simulink model "test_equalizer"  (Simulink 7.4)
settings: Solver=ode45  StartTime=0  StopTime=100  RelTol=1e-3
libraries: xbsIndex_r4 x7, casper_library x2, xps_library x1, isi_correlator_lib x1
settings Model: Creator=wjm  LastModifiedBy=wjm
settings OptimizationCC: InitFltsAndDblsToZero=on

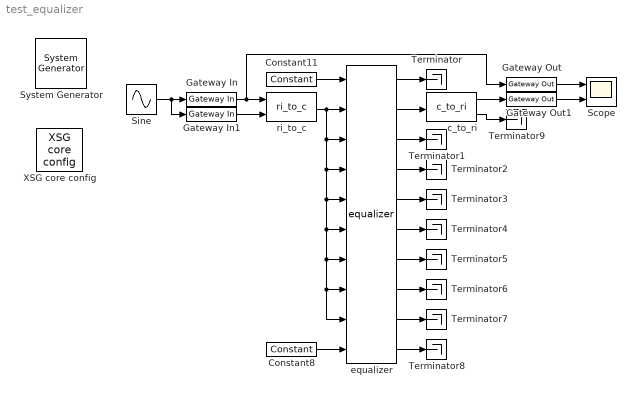
== system test_equalizer ==
  " System Generator" : xbsIndex_r4/ System Generator  Tag=genX  SystemSampleTime=-1  xilinxfamily=virtex5  part=xc5vsx95t  speed=-1  package=ff1136  synthesis_tool=XST  clock_wrapper=Clock Enables  directory=./isi_spectrometer/sysgen  testbench=off  simulink_period=1  sysclk_period=5  dcm_input_clock_period=100  incr_netlist=off  trim_vbits=Everywhere in SubSystem  dbl_ovrd=According to Block Masks  core_generation=According to Block Masks  run_coregen=off  deprecated_control=off  eval_field=0  block_type=sysgen
      settings: block_version=10.1.1
  Constant11 : xbsIndex_r4/Constant  arith_type=Boolean  const=0  n_bits=1  bin_pt=0  explicit_period=on  period=1  equ=P=C  opselect=C  inp2=PCIN>>17  opr=+  inp1=P  carry=CIN  dbl_ovrd=off  block_type=constant
      settings: block_version=10.1.1
  Constant8 : xbsIndex_r4/Constant  arith_type=Unsigned  const=1  n_bits=4  bin_pt=0  explicit_period=on  period=1  equ=P=C  opselect=C  inp2=PCIN>>17  opr=+  inp1=P  carry=CIN  dbl_ovrd=off  block_type=constant
      settings: block_version=10.1.1
  Gateway In : xbsIndex_r4/Gateway In  arith_type="Signed  (2's comp)"  n_bits=8  bin_pt=7  quantization="Round  (unbiased: +/- Inf)"  overflow=Wrap  period=1  dbl_ovrd=off  timing_constraint=None  locs_specified=off  LOCs={}  hdl_port=on  block_type=gatewayin
      settings: infoedit="Gateway in block.  Converts inputs of type Simulink integer, double and fixed point to  Xilinx fixed point type.<br><br>Hardware notes:  In hardware these blocks become top level input ports."  block_version=10.1.3
  Gateway In1 : xbsIndex_r4/Gateway In  arith_type="Signed  (2's comp)"  n_bits=8  bin_pt=7  quantization=Truncate  overflow=Wrap  period=1  dbl_ovrd=off  timing_constraint=None  locs_specified=off  LOCs={}  hdl_port=on  block_type=gatewayin
      settings: infoedit="Gateway in block.  Converts inputs of type Simulink integer, double and fixed point to  Xilinx fixed point type.<br><br>Hardware notes:  In hardware these blocks become top level input ports."  block_version=10.1.3
  Gateway Out : xbsIndex_r4/Gateway Out  hdl_port=on  timing_constraint=None  locs_specified=off  LOCs={}  block_type=gatewayout
      settings: infoedit="Gateway out block.  Converts Xilinx fixed point inputs into ouputs of type Simulink integer, double, or fixed point.<P><P>Hardware notes:  In hardware these blocks become top level output ports or are discarded, depending on how they are configured."  block_version=10.1.3
  Gateway Out1 : xbsIndex_r4/Gateway Out  hdl_port=on  timing_constraint=None  locs_specified=off  LOCs={}  block_type=gatewayout
      settings: infoedit="Gateway out block.  Converts Xilinx fixed point inputs into ouputs of type Simulink integer, double, or fixed point.<P><P>Hardware notes:  In hardware these blocks become top level output ports or are discarded, depending on how they are configured."  block_version=10.1.3
  Scope : Scope  NumInputPorts=2
      settings: YMin=-5~-5  YMax=5~5
  Sine : Sin  Amplitude=7/8  Bias=0  Frequency=10*(2*pi/375)  Phase=0  Samples=10  SampleTime=1  Offset=0
  Terminator{,1..9} (10 alike) : Terminator
  XSG core config : xps_library/XSG core config  Tag=xps:xsg  SystemSampleTime=-1  hw_sys=ROACH:sx95t  ibob_linux=off  clk_src=adc0_clk  iBOB_clk_src=sys_clk  BEE2_ctrl_clk_src=sys_clk  BEE2_usr_clk_src=sys_clk  ROACH_clk_src=adc0_clk  CORR_clk_src=sys_clk  gpio_clk_io_group=iBOB:sma  gpio_clk_bit_index=0  clk_rate=200  sample_period=1  synthesis_tool=XST  mpc_type=powerpc440_ext
  c_to_ri : casper_library/Misc/c_to_ri  SystemSampleTime=-1  n_bits=4  bin_pt=3
      settings: AttributesFormatString=4_3 r/i
  equalizer : isi_correlator_lib/equalizer  SystemSampleTime=-1  in_bit_width=8  out_bit_width=4
      link override scale0/saturate_real/Convert: arith_type="Signed  (2's comp)"  n_bits=dout_bit_width  bin_pt=dout_bit_width - 1  quantization="Round  (unbiased: Even Values)"  overflow=Wrap  latency=2  dbl_ovrd=off  pipeline=off
      link override scale0/saturate_real/Convert: infoedit=Hardware notes: rounding and saturating require hardware resources; truncating and wrapping do not.
  ri_to_c : casper_library/Misc/ri_to_c  SystemSampleTime=-1
  wires:
  Constant11/1 -> equalizer/1
  equalizer/1 -> Terminator/1
  equalizer/3 -> Terminator1/1
  equalizer/4 -> Terminator2/1
  equalizer/5 -> Terminator3/1
  equalizer/6 -> Terminator4/1
  equalizer/7 -> Terminator5/1
  equalizer/8 -> Terminator6/1
  equalizer/9 -> Terminator7/1
  equalizer/10 -> Terminator8/1
  Sine/1 -> Gateway In/1, Gateway In1/1
  Gateway In/1 -> ri_to_c/1, Gateway Out/1
  Gateway In1/1 -> ri_to_c/2
  ri_to_c/1 -> equalizer/2, equalizer/3, equalizer/4, equalizer/5, equalizer/6, equalizer/7, equalizer/9, equalizer/8
  equalizer/2 -> c_to_ri/1
  Gateway Out/1 -> Scope/1
  Gateway Out1/1 -> Scope/2
  Constant8/1 -> equalizer/10
  c_to_ri/1 -> Gateway Out1/1
  c_to_ri/2 -> Terminator9/1
